simulink model "OFDMTxRx2211"  (R2017b)
settings: Solver=VariableStepAuto  StartTime=0.0  StopTime=10.0  RelTol=1e-3
InitFcn:
  | Ts = 1e-6;
  | simParams.Ts = Ts;
  | simParams.TsTx = Ts;
  | simParams.TsRx = Ts;
  | simParams.nFFT = 1024;
  | simParams.lengthCP = 128;
  | nFFT = simParams.nFFT;
  | simParams.NSubcarriers = 398;
  | simParams.windowing = 16;
undefined symbols (not defined in the file): fft_size, i
libraries: hdlsllib x49, simulink x39, simulink_need_slupdate x12, dspmathops x4, dspxfrm3 x3, dspsigops x2, commdigbbndam3 x1, commseqgen3 x1
(part 3 of 3)

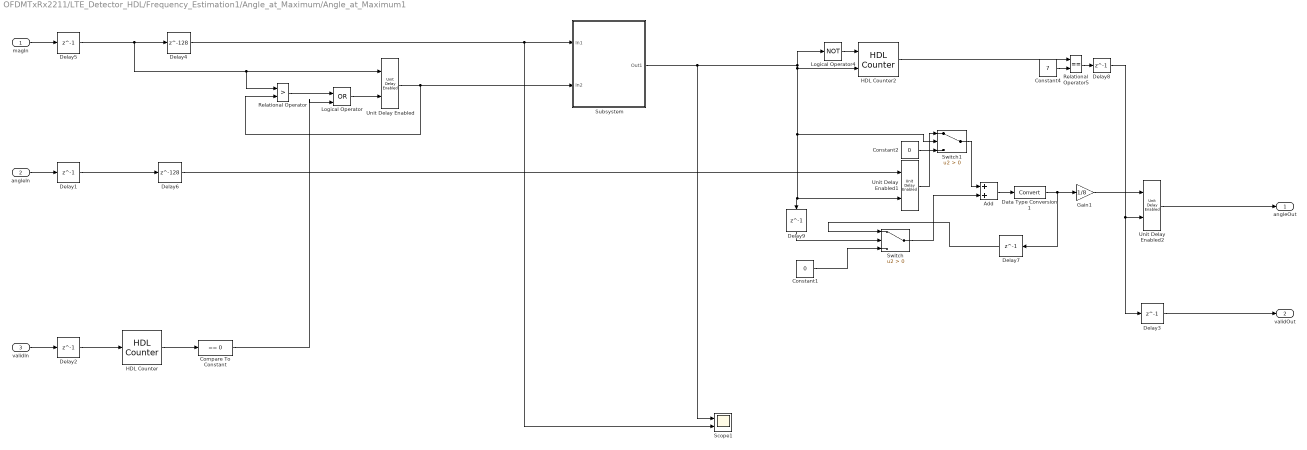
== system OFDMTxRx2211/LTE_Detector_HDL/Frequency_Estimation1/Angle_at_Maximum/Angle_at_Maximum1 ==
  magIn : Inport
  angleIn : Inport  Port=2
  validIn : Inport  Port=3
  Add : Sum
  Compare To Constant : simulink/Logic and Bit Operations/Compare To Constant  relop===  const=0  OutDataTypeStr=boolean
  Constant1 : Constant  Value=0
  Constant2 : Constant  Value=0
  Constant4 : Constant  Value=7
  Data Type Conversion1 : DataTypeConversion
  Delay{1..3,5,7..9} (7 alike) : Delay  DelayLength=1  InitialCondition=0  UseCircularBuffer=on
  Delay4 : Delay  DelayLength=128  InitialCondition=0  UseCircularBuffer=on
  Delay6 : Delay  DelayLength=128  InitialCondition=0  UseCircularBuffer=on
  Gain1 : Gain  Gain=1/8
  HDL Counter : hdlsllib/Sources/HDL Counter  CountType=Count limited  CountInit=0  CountStep=1  CountMax=1152  CountFromType=Initial value  CountFrom=0  CountResetPort=off  CountLoadPort=off  CountEnbPort=on  CountDirPort=off  CountDataType=Unsigned  CountWordLen=11  CountFracLen=0  CountSampTime=1
      settings: SourceProductBaseCode=HD
  HDL Counter2 : hdlsllib/Sources/HDL Counter  CountType=Count limited  CountInit=0  CountStep=1  CountMax=7  CountFromType=Initial value  CountFrom=0  CountResetPort=on  CountLoadPort=off  CountEnbPort=on  CountDirPort=off  CountDataType=Unsigned  CountWordLen=3  CountFracLen=0  CountSampTime=1
      settings: SourceProductBaseCode=HD
  Logical Operator : Logic  Operator=OR  IconShape=distinctive  AllPortsSameDT=off  OutDataTypeStr=boolean
  Logical Operator4 : Logic  Operator=NOT  IconShape=distinctive  AllPortsSameDT=off  OutDataTypeStr=boolean
  Relational Operator : RelationalOperator  Operator=>  OutDataTypeStr=boolean  RndMeth=Nearest
  Relational Operator5 : RelationalOperator  Operator===  OutDataTypeStr=boolean  RndMeth=Nearest
  Scope1 : Scope  NumInputPorts=2
  Subsystem : Subsystem
  Switch : Switch  Criteria=u2 > Threshold
  Switch1 : Switch  Criteria=u2 > Threshold
  Unit Delay Enabled : simulink_need_slupdate/Unit Delay Enabled  vinit=0.0  tsamp=-1
      settings: SourceProductName=Simulink  SourceProductBaseCode=SL
  Unit Delay Enabled1 : simulink_need_slupdate/Unit Delay Enabled  vinit=0.0  tsamp=-1
      settings: SourceProductName=Simulink  SourceProductBaseCode=SL
  Unit Delay Enabled2 : simulink_need_slupdate/Unit Delay Enabled  vinit=0.0  tsamp=-1
      settings: SourceProductName=Simulink  SourceProductBaseCode=SL
  angleOut : Outport
  validOut : Outport  Port=2
  wires:
  magIn/1 -> Delay5/1
  angleIn/1 -> Delay1/1
  HDL Counter/1 -> Compare To Constant/1
  Compare To Constant/1 -> Logical Operator/2
  validIn/1 -> Delay2/1
  Delay5/1 -> Relational Operator/1, Unit Delay Enabled/1, Delay4/1
  Delay2/1 -> HDL Counter/1
  Unit Delay Enabled/1 -> Subsystem/2(In2), Relational Operator/2
  Relational Operator/1 -> Logical Operator/1
  Logical Operator/1 -> Unit Delay Enabled/2
  Delay1/1 -> Delay6/1
  Delay6/1 -> Unit Delay Enabled1/1
  Add/1 -> Data Type Conversion1/1
  Constant4/1 -> Relational Operator5/2
  HDL Counter2/1 -> Relational Operator5/1
  Relational Operator5/1 -> Delay8/1
  Unit Delay Enabled2/1 -> angleOut/1
  Logical Operator4/1 -> HDL Counter2/1
  Subsystem/1(Out1) -> Scope1/1, Switch1/2, Delay9/1, Unit Delay Enabled1/2, HDL Counter2/2, Logical Operator4/1
  Delay4/1 -> Scope1/2, Subsystem/1(In1)
  Gain1/1 -> Unit Delay Enabled2/1
  Delay7/1 -> Switch/1
  Data Type Conversion1/1 -> Delay7/1, Gain1/1
  Constant1/1 -> Switch/3
  Switch/1 -> Add/2
  Delay9/1 -> Switch/2
  Constant2/1 -> Switch1/3
  Unit Delay Enabled1/1 -> Switch1/1
  Switch1/1 -> Add/1
  Delay8/1 -> Unit Delay Enabled2/2, Delay3/1
  Delay3/1 -> validOut/1

== system OFDMTxRx2211/LTE_Detector_HDL/Frequency_Estimation1/Cyclic_Prefix_Correlator/Moving_Average ==
  note: Use a comb filter followed by an integrator
      | to implement an efficient 9-tab moving average.
  dataIn : Inport
  Add : Sum  Inputs=-+  AccumDataTypeStr=fixdt(1,27,23)
  Add1 : Sum  AccumDataTypeStr=fixdt(1,27,23)
  Delay1 : Delay  DelayLength=128  InitialCondition=0
  Delay10 : Delay  DelayLength=1  InitialCondition=0  UseCircularBuffer=on
  Delay2 : Delay  DelayLength=1  InitialCondition=0  UseCircularBuffer=on
  Delay3 : Delay  DelayLength=1  InitialCondition=0  UseCircularBuffer=on
  Gain : Gain  Gain=1/128  OutDataTypeStr=fixdt(1,24,23)
  dataOut : Outport
  wires:
  dataIn/1 -> Add/2, Delay1/1
  Delay1/1 -> Add/1
  Add1/1 -> Delay2/1
  Delay10/1 -> Add1/2
  Delay2/1 -> Gain/1, Add1/1
  Delay3/1 -> dataOut/1
  Gain/1 -> Delay3/1
  Add/1 -> Delay10/1

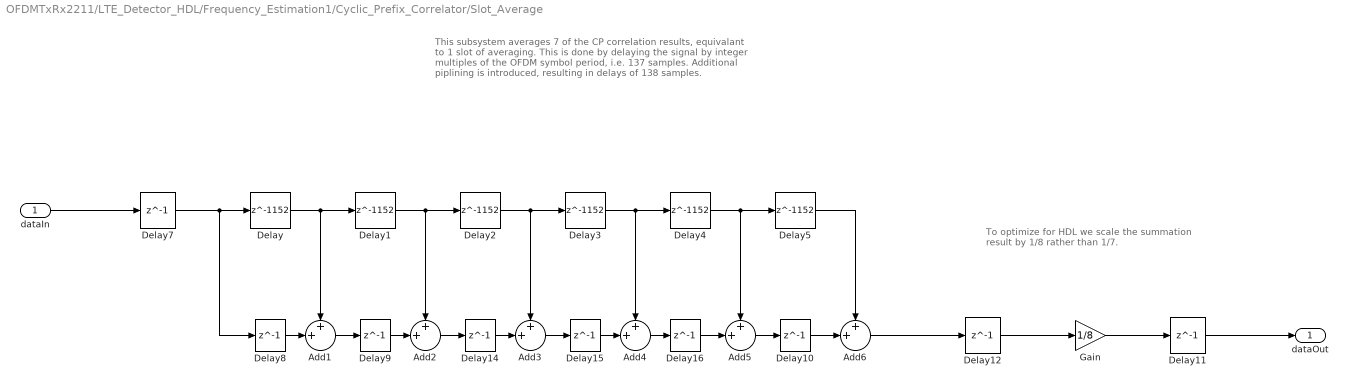
== system OFDMTxRx2211/LTE_Detector_HDL/Frequency_Estimation1/Cyclic_Prefix_Correlator/Slot_Average ==
  note: This subsystem averages 7 of the CP correlation results, equivalant to 1 slot of averaging. This is done by delaying the signal by integer multiples of the OFDM symbol period, i.e. 137 samples.
      |
      | Additional piplining is introduced, resulting in delays of 138 samples.
  note: To optimize for HDL we scale the summation result by 1/8 rather than 1/7.
  dataIn : Inport
  Add1 : Sum  Inputs=++|  AccumDataTypeStr=fixdt(1,28,23)
  Add2 : Sum  Inputs=++|  AccumDataTypeStr=fixdt(1,29,23)
  Add3 : Sum  Inputs=++|  OutDataTypeStr=fixdt(1,29,23)
  Add4 : Sum  Inputs=++|  AccumDataTypeStr=fixdt(1,29,23)
  Add5 : Sum  Inputs=++|  AccumDataTypeStr=fixdt(1,30,23)
  Add6 : Sum  Inputs=++|  AccumDataTypeStr=fixdt(1,30,23)
  Delay{,1..5} (6 alike) : Delay  DelayLength=1152  InitialCondition=0
  Delay{7..12,14..16} (9 alike) : Delay  DelayLength=1  InitialCondition=0  UseCircularBuffer=on
  Gain : Gain  Gain=1/8  OutDataTypeStr=fixdt(1,24,23)
  dataOut : Outport
  wires:
  Delay4/1 -> Delay5/1, Add5/1
  Delay/1 -> Delay1/1, Add1/1
  Add1/1 -> Delay9/1
  Delay1/1 -> Delay2/1, Add2/1
  Delay3/1 -> Delay4/1, Add4/1
  Delay2/1 -> Delay3/1, Add3/1
  dataIn/1 -> Delay7/1
  Add2/1 -> Delay14/1
  Add3/1 -> Delay15/1
  Add4/1 -> Delay16/1
  Add5/1 -> Delay10/1
  Delay5/1 -> Add6/1
  Add6/1 -> Delay12/1
  Delay7/1 -> Delay8/1, Delay/1
  Delay8/1 -> Add1/2
  Delay9/1 -> Add2/2
  Delay14/1 -> Add3/2
  Delay15/1 -> Add4/2
  Delay16/1 -> Add5/2
  Delay10/1 -> Add6/2
  Delay12/1 -> Gain/1
  Gain/1 -> Delay11/1
  Delay11/1 -> dataOut/1

== system OFDMTxRx2211/LTE_Detector_HDL/Frequency_Estimation/Angle_at_Maximum/Нахождение окрестности середины ЗИ/Задержка максимального значения ==
  AmpIn : Inport
  "Reset " : Inport  Port=2
  Logical Operator : Logic  Operator=OR  IconShape=distinctive  AllPortsSameDT=off  OutDataTypeStr=boolean
  Relational Operator : RelationalOperator  Operator=>  OutDataTypeStr=boolean  RndMeth=Nearest
  Unit Delay Enabled : simulink_need_slupdate/Unit Delay Enabled  vinit=0.0  tsamp=-1
      settings: SourceProductName=Simulink  SourceProductBaseCode=SL
  Out1 : Outport
  wires:
  Logical Operator/1 -> Unit Delay Enabled/2
  Unit Delay Enabled/1 -> Out1/1, Relational Operator/2
  Relational Operator/1 -> Logical Operator/1
  "Reset "/1 -> Logical Operator/2
  AmpIn/1 -> Relational Operator/1, Unit Delay Enabled/1

== system OFDMTxRx2211/LTE_Detector_HDL/Frequency_Estimation1/Angle_at_Maximum/Angle_at_Maximum1/Subsystem ==
  In1 : Inport
  In2 : Inport  Port=2
  Constant : Constant  Value=4.5*10^-4
  Constant1 : Constant  Value=60
  Constant2 : Constant  Value=67
  Gain : Gain  Gain=0.7
  HDL Counter1 : hdlsllib/Sources/HDL Counter  CountType=Count limited  CountInit=0  CountStep=1  CountMax=1152  CountFromType=Initial value  CountFrom=0  CountResetPort=on  CountLoadPort=off  CountEnbPort=on  CountDirPort=off  CountDataType=Unsigned  CountWordLen=11  CountFracLen=0  CountSampTime=1
      settings: SourceProductBaseCode=HD
  Logical Operator1 : Logic  IconShape=distinctive  AllPortsSameDT=off  OutDataTypeStr=boolean
  Logical Operator2 : Logic  Operator=NOT  IconShape=distinctive  AllPortsSameDT=off  OutDataTypeStr=boolean
  Logical Operator3 : Logic  IconShape=distinctive  AllPortsSameDT=off  OutDataTypeStr=boolean
  Relational Operator1 : RelationalOperator  Operator=>  OutDataTypeStr=boolean  RndMeth=Nearest
  Relational Operator2 : RelationalOperator  Operator=>  OutDataTypeStr=boolean  RndMeth=Nearest
  Relational Operator3 : RelationalOperator  OutDataTypeStr=boolean  RndMeth=Nearest
  Relational Operator4 : RelationalOperator  Operator=<=  OutDataTypeStr=boolean  RndMeth=Nearest
  Out1 : Outport
  wires:
  In2/1 -> Gain/1
  Gain/1 -> Relational Operator1/2
  Logical Operator1/1 -> Logical Operator2/1, HDL Counter1/2
  Relational Operator1/1 -> Logical Operator1/2
  Logical Operator2/1 -> HDL Counter1/1
  Constant/1 -> Relational Operator2/2
  Relational Operator2/1 -> Logical Operator1/1
  Constant1/1 -> Relational Operator3/2
  In1/1 -> Relational Operator2/1, Relational Operator1/1
  HDL Counter1/1 -> Relational Operator4/1, Relational Operator3/1
  Relational Operator3/1 -> Logical Operator3/1
  Constant2/1 -> Relational Operator4/2
  Relational Operator4/1 -> Logical Operator3/2
  Logical Operator3/1 -> Out1/1
